simulink model "RaspiGreenBall"  (R2014a)
settings: Solver=FixedStepDiscrete  StartTime=0.0  StopTime=10.0  RelTol=1e-3
libraries: embdlinuxlib x2, visionstatistics x1, visiontextngfix x1
settings Model: ExtModeTrigDuration=100  Creator=akaushik  LastModifiedBy=yanlianz
settings OptimizationCC: OptimizeModelRefInitCode=on  LifeSpan=1
settings DebuggingCC: UnderspecifiedInitializationDetection=Classic  SolverPrmCheckMsg=none
settings HardwareCC: ProdLargestAtomicInteger=Long  ProdLargestAtomicFloat=Double  ProdEndianess=LittleEndian  ProdHWDeviceType=ARM Compatible->ARM Cortex
settings RTWCC: SystemTargetFile=realtime.tlc  GenerateMakefile=off  TemplateMakefile=realtime.tmf  Description=Run on Target Hardware  RTWVerbose=off  ProcessScript=realtime_make_rtw_hook
settings STFCustomTargetCC: TargetLibSuffix=.a  GenerateSampleERTMain=on  ConcurrentExecutionCompliant=off  GeneratePreprocessorConditionals=Use local settings  ERTCustomFileBanners=on  SupportNonInlinedSFcns=off  SupportVariableSizeSignals=on  MATLABClassNameForMDSCustomization=Simulink.SoftwareTarget.ERTCustomization  GRTInterface=off  SystemTargetFile=realtime.tlc
settings ERTTargetCC: CombineOutputUpdateFcns=off  SupportContinuousTime=on  SupportVariableSizeSignals=on  ExtModeMexArgs='172.28.138.195' 0 17725  ERTSrcFileBannerTemplate=realtime_code_template.cgt  ERTHdrFileBannerTemplate=realtime_code_template.cgt  ERTDataSrcFileTemplate=realtime_code_template.cgt  ERTDataHdrFileTemplate=realtime_code_template.cgt  ERTCustomFileTemplate=realtime_file_process.tlc

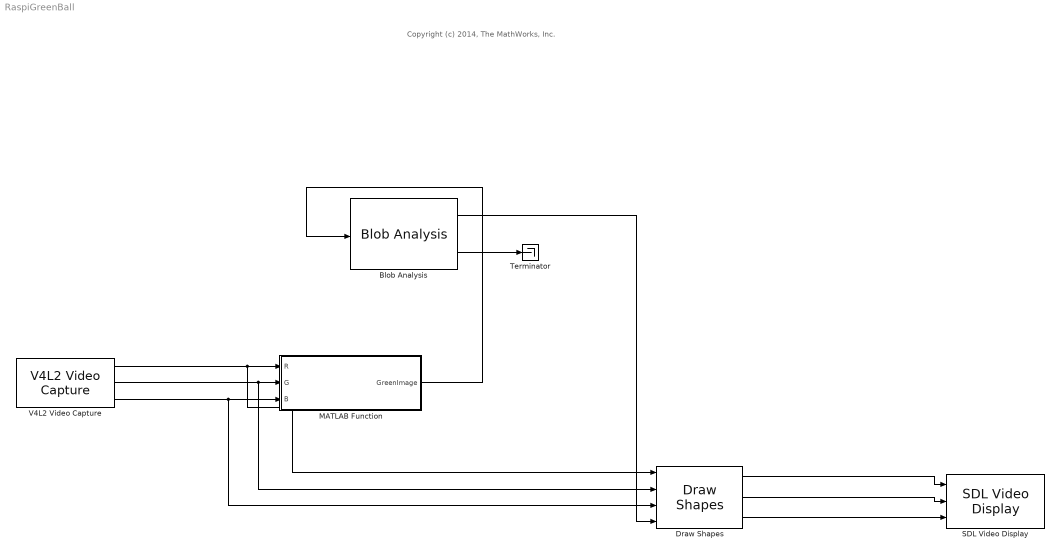
== system RaspiGreenBall ==
  note: Copyright (c) 2014, The MathWorks, Inc.
  Blob Analysis : visionstatistics/Blob Analysis  Tag=vipblks_row_conv  area=off  centroid=off  bBox=on  majorAxis=off  minorAxis=off  angle=off  eccentricity=off  equivDiameterSq=off  extent=off  perimeter=off  maxBlobs=1  warnIfNumBlobsExceeded=off  isCount=on  useMinArea=on  minArea=300  useMaxArea=off  maxArea=intmax('uint32')  excludeBorderBlob=on  outDT=double  isOutVarDim=off  isFill=on  fillValues=-1  conn=8  isLabel=off  outputMode=Binary point scaling  outputWordLength=32  outputFracLength=16  firstCoeffMode=Binary point scaling  firstCoeffWordLength=16  firstCoeffFracLength=14  secondCoeffMode=Binary point scaling  secondCoeffWordLength=32  secondCoeffFracLength=16  accumMode=Binary point scaling  accumWordLength=32  accumFracLength=0  prodOutputMode=Binary point scaling  prodOutputWordLength=32  prodOutputFracLength=16  roundingMode=Floor  overflowMode=off
  Draw Shapes : visiontextngfix/Draw Shapes  shape=Rectangles  fill=off  lineWidth=1  fillClrSource=Specify via dialog  display=White  intensity=200  color=[200 255 100]  opacity=0.6  viewport=Entire image  antialiasing=off  inType=Obsolete  imagePorts=Separate color signals  prodOutputMode=Binary point scaling  prodOutputWordLength=32  prodOutputFracLength=14  memoryMode=Specify word length  memoryWordLength=16  memoryFracLength=15  roundingMode=Floor  overflowMode=off
  MATLAB Function : MATLAB Function  TreatAsAtomicUnit=on
  SDL Video Display : embdlinuxlib/SDL Video Display  pixelFormat=RGB  pixelOrder=Planar  rowMajor=on  blockPlatform=Raspberry Pi
  Terminator : Terminator
  V4L2 Video Capture : embdlinuxlib/V4L2 Video Capture  m_devName='/dev/video0'  roi=[0, 0, 640, 480]  imSizeSelection=320x240  imSize=[640, 480]  pixelFormat=RGB  pixelOrder=Planar  sampleTime=1/30  simOutput=Colorbars  blockPlatform=Raspberry Pi
  wires:
  Draw Shapes/2 -> SDL Video Display/2
  Draw Shapes/3 -> SDL Video Display/3
  Blob Analysis/1 -> Draw Shapes/4
  Draw Shapes/1 -> SDL Video Display/1
  MATLAB Function/1(GreenImage) -> Blob Analysis/1
  V4L2 Video Capture/1 -> Draw Shapes/1, MATLAB Function/1(R)
  V4L2 Video Capture/2 -> Draw Shapes/2, MATLAB Function/2(G)
  V4L2 Video Capture/3 -> Draw Shapes/3, MATLAB Function/3(B)
  Blob Analysis/2 -> Terminator/1

== matlab function RaspiGreenBall/MATLAB Function ==
  data: R input; GreenImage output; G input; B input
function GreenImage = ColorThresholding(R,G,B)
%#codegen


I = 3*G - 2*R - 2*B;
GreenImage = ~(I < 0.9);

end
